simulink model "sus_auto_ulink"  (R2024a)
settings: Solver=VariableStepAuto  StartTime=0.0  StopTime=10.0  RelTol=1e-3
model workspace (MAT data in the model file):
  b = Simulink.Parameter
  b.Value = 1000
  b.Complexity = 'real'
  b.Dimensions = [1 1]
  b.DataType = 'auto'
  k1 = Simulink.Parameter
  k1.Value = 16182
  k1.Complexity = 'real'
  k1.Dimensions = [1 1]
  k1.DataType = 'auto'
  k2 = Simulink.Parameter
  k2.Value = 19000
  k2.Complexity = 'real'
  k2.Dimensions = [1 1]
  k2.DataType = 'auto'
  m1 = Simulink.Parameter
  m1.Value = 290
  m1.Complexity = 'real'
  m1.Dimensions = [1 1]
  m1.DataType = 'auto'
  m2 = Simulink.Parameter
  m2.Value = 59
  m2.Complexity = 'real'
  m2.Dimensions = [1 1]
  m2.DataType = 'auto'
values from neighbouring files (symbols this model uses):
  b = 1000    [sus_auto.m]
  k1 = 16182    [sus_auto.m]
  k2 = 19000    [sus_auto.m]
  m1 = 290    [sus_auto.m]
  m2 = 59    [sus_auto.m]
settings Model: Creator=JUAN CARLOS  LastModifiedBy=JUAN CARLOS

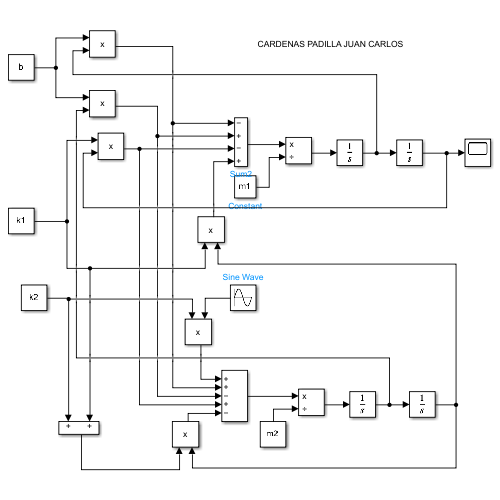
[thumbnail: Simulink's stored preview of the top-level diagram]
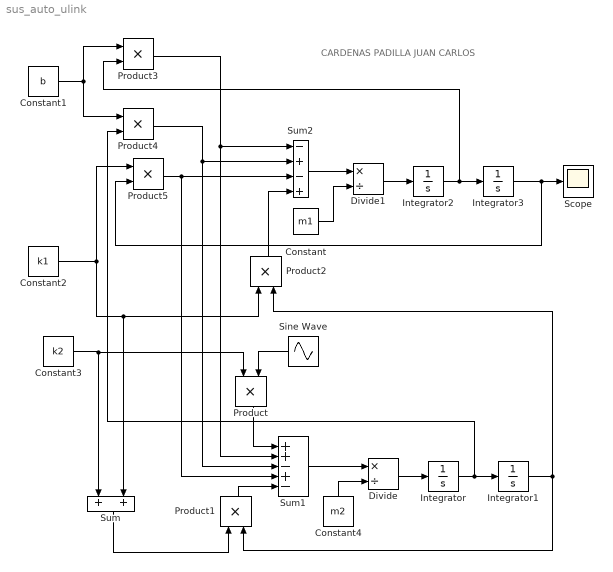
== system sus_auto_ulink ==
  note: CARDENAS PADILLA JUAN CARLOS
  Constant : Constant  Value=m1
  Constant1 : Constant  Value=b
  Constant2 : Constant  Value=k1
  Constant3 : Constant  Value=k2
  Constant4 : Constant  Value=m2
  Divide : Product  Inputs=*/
  Divide1 : Product  Inputs=*/
  Integrator{,1..3} (4 alike) : Integrator
  Product{,1..5} (6 alike) : Product
  Scope : Scope
  Sine Wave : Sin  Amplitude=0.05  Frequency=0.5*pi  SampleTime=0
  Sum : Sum
  Sum1 : Sum  Inputs=++-+-
  Sum2 : Sum  Inputs=-+-+
  wires:
  Constant3/1 -> Sum/1, Product/1
  Sine Wave/1 -> Product/2
  Sum/1 -> Product1/1
  Product1/1 -> Sum1/5
  Product/1 -> Sum1/1
  Sum1/1 -> Divide/1
  Divide/1 -> Integrator/1
  Integrator/1 -> Product4/2, Integrator1/1
  Integrator1/1 -> Product1/2, Product2/2
  Constant4/1 -> Divide/2
  Constant2/1 -> Sum/2, Product2/1, Product5/1
  Product2/1 -> Sum2/4
  Constant/1 -> Divide1/2
  Sum2/1 -> Divide1/1
  Constant1/1 -> Product4/1, Product3/1
  Divide1/1 -> Integrator2/1
  Integrator2/1 -> Integrator3/1, Product3/2
  Integrator3/1 -> Product5/2, Scope/1
  Product3/1 -> Sum2/1, Sum1/2
  Product4/1 -> Sum2/2, Sum1/3
  Product5/1 -> Sum2/3, Sum1/4
